simulink model "Particle_Formation"  (R2024b)
settings: Solver=VariableStepAuto  StartTime=0.0  StopTime=300  RelTol=1e-3
settings Model: Creator=Omar  LastModifiedBy=Omar
settings SolverCC: ZeroCrossAlgorithm=Adaptive
settings DebuggingCC: IgnoredZcDiagnostic=none

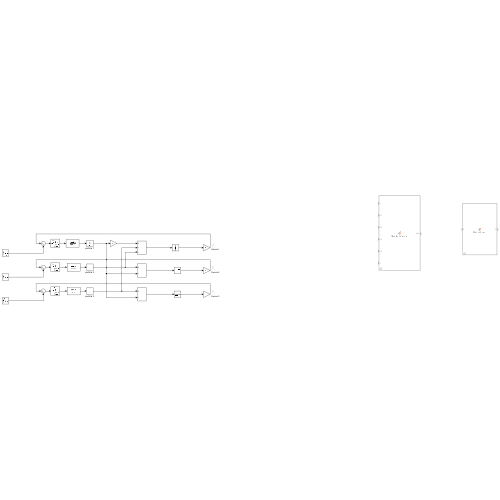
[thumbnail: Simulink's stored preview of the top-level diagram]
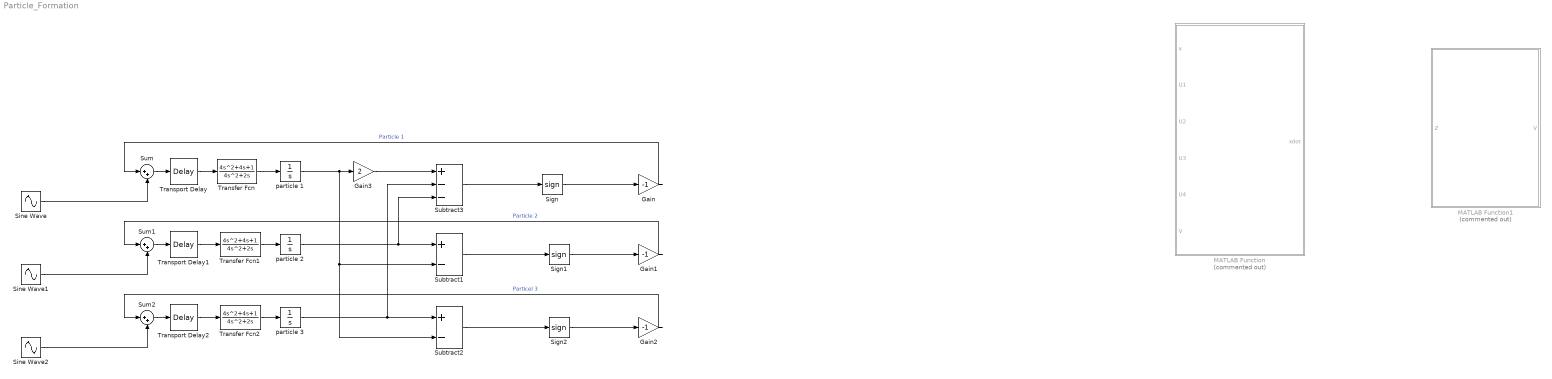
== system Particle_Formation ==
  Gain : Gain  Gain=-1
  Gain1 : Gain  Gain=-1
  Gain2 : Gain  Gain=-1
  Gain3 : Gain  Gain=2
  MATLAB Function : MATLAB Function  Commented=on  TreatAsAtomicUnit=on
  MATLAB Function1 : MATLAB Function  Commented=on  TreatAsAtomicUnit=on
  Sign : Signum
  Sign1 : Signum
  Sign2 : Signum
  Sine Wave : Sin  SampleTime=0
  Sine Wave1 : Sin  SampleTime=0
  Sine Wave2 : Sin  SampleTime=0
  Subtract1 : Sum  Inputs=+-
  Subtract2 : Sum  Inputs=+-
  Subtract3 : Sum  Inputs=+--
  Sum : Sum  Inputs=|++
  Sum1 : Sum  Inputs=|++
  Sum2 : Sum  Inputs=|++
  Transfer Fcn : TransferFcn  Numerator=[4 4 1]  Denominator=[4 2 0]
  Transfer Fcn1 : TransferFcn  Numerator=[4 4 1]  Denominator=[4 2 0]
  Transfer Fcn2 : TransferFcn  Numerator=[4 4 1]  Denominator=[4 2 0]
  Transport Delay : TransportDelay  DelayTime=2
  Transport Delay1 : TransportDelay  DelayTime=2
  Transport Delay2 : TransportDelay  DelayTime=2
  particle 1 : Integrator  InitialCondition=20
  particle 2 : Integrator  InitialCondition=1
  particle 3 : Integrator  InitialCondition=50
  wires:
  Sign2/1 -> Gain2/1
  Subtract2/1 -> Sign2/1
  Subtract1/1 -> Sign1/1
  Sign1/1 -> Gain1/1
  Gain2/1 -> Sum2/1  "Particel 3"
  particle 1/1 -> Subtract2/2, Subtract1/2, Gain3/1
  Subtract3/1 -> Sign/1
  Sign/1 -> Gain/1
  Sine Wave/1 -> Sum/2
  Sine Wave1/1 -> Sum1/2
  Sine Wave2/1 -> Sum2/2
  particle 2/1 -> Subtract3/3, Subtract1/1
  particle 3/1 -> Subtract3/2, Subtract2/1
  Gain/1 -> Sum/1  "Particle 1"
  Gain3/1 -> Subtract3/1
  Gain1/1 -> Sum1/1  "Particle 2"
  Sum/1 -> Transport Delay/1
  Sum1/1 -> Transport Delay1/1
  Sum2/1 -> Transport Delay2/1
  Transfer Fcn1/1 -> particle 2/1
  Transport Delay2/1 -> Transfer Fcn2/1
  Transfer Fcn2/1 -> particle 3/1
  Transport Delay1/1 -> Transfer Fcn1/1
  Transport Delay/1 -> Transfer Fcn/1
  Transfer Fcn/1 -> particle 1/1

== matlab function Particle_Formation/MATLAB Function1 ==
  data: Z input; V output
function V  = RotorModel(Z)

V = zeros(4,1);
V(1) = Z(1)^2/2;
V(2) = (V(1) + Z(2)^2)/2;
V(3) = Z(3)^2/2;
V(4) = (V(3) + Z(4)^2)/2;

== matlab function Particle_Formation/MATLAB Function ==
  data: x input; xdot output; U1 input; U2 input; U3 input; U4 input; V input
function xdot = QuadrotorModel(x, U1, U2, U3, U4, V)
% x = (phi p theta q psi r x xdot y ydot z zdot)

%omega_bar = w1-w2+w3-w4
omega_bar = x(13) - x(14) + x(15) - x(16);
b = 280.19; beta0 = 189.63; beta1 = 6.0612; beta2 = 0.0122;

%initializing constants
m = 1.029; g = 9.81;
Ix = 15.48835e-3; Iy = Ix; Iz = 22.5656e-3;
Jr = 2.8385e-5;
% Jr = 0.0;
al = (Iy-Iz)/Ix; a3 = -Jr/Ix;
a4 = (Iz-Ix)/Iy; a6 = Jr/Iy;
a7 = (Ix-Iy)/Iz;
b1 = 1.1/Ix; b2 = 1.1/Iy; b3 = 0.2/Iz;
Ux = cos(x(1)) * sin(x(3)) * cos(x(5)) + sin(x(1)) * sin(x(5));
Uy = cos(x(1)) * sin(x(3)) * sin(x(5)) - sin(x(1)) * cos(x(5));
Uz = cos(x(1)) * cos(x(3));

% Introduce parameter uncertainty and distrubances
% Weak and Heavy Model:
% m = 1.2*m; U1 = 0.8*U1;
% Strong and Light Model:
% m = 0.8*m; U1 = 1.2*U1;

%Dynamics of the quadrotor
xdot = zeros(16,1);
xdot(1) = x(2) + x(4)*sin(x(1))*tan(x(3)) + x(6)*cos(x(1))*tan(x(3));
xdot(2) = al*x(4)*x(6) + a3*omega_bar*x(4) + b1*U2;
xdot(3) = x(4)*cos(x(1)) - x(6)*sin(x(1));
xdot(4) = a4*x(2)*x(6) + a6*omega_bar*x(2) + b2*U3;
xdot(5) = x(6)*(cos(x(1))/cos(x(3))) + x(4)*(sin(x(1))/cos(x(3)));
xdot(6) = a7*x(2)*x(4) + b3*U4;
xdot(7) = x(8);
xdot(8) = (Ux*U1)/m;
xdot(9) = x(10);
xdot(10) = (Uy*U1)/m;
xdot(11) = x(12);
xdot(12) = (Uz*U1)/m - g;
xdot(13) = b*V(1) - beta0 - beta1*x(13) - beta2*x(13)^2;
xdot(14) = b*V(2) - beta0 - beta1*x(14) - beta2*x(14)^2;
xdot(15) = b*V(3) - beta1 - beta1*x(15) - beta2*x(15)^2;
xdot(16) = b*V(4) - beta1 - beta1*x(16) - beta2*x(16)^2;
